simulink model "OldCameraGantryStuff"  (Simulink 7.8)
settings: Solver=FixedStepDiscrete  SolverMode=SingleTasking  StartTime=0.0  StopTime=5.659  FixedStep=0.001  RelTol=1e-3
values from neighbouring files (symbols this model uses):
  T_step = 0.01    [CoefficientsForFilters.mat]    (also in matlab.mat = 0.001)
undefined symbols (not defined in the file or in its folder): DiscIntNeverNeededParam
settings Model: Creator=Marx  LastModifiedBy=root
settings OptimizationCC: OptimizeModelRefInitCode=on  LifeSpan=1
settings HardwareCC: ProdBitPerInt=16  ProdBitPerPointer=16  ProdEndianess=LittleEndian  ProdWordSize=16  ProdHWDeviceType=16-bit Generic
settings RTWCC: SystemTargetFile=dspic.tlc  GenCodeOnly=on  MakeCommand=make_CreateMPLAB  TemplateMakefile=dspic_pic30_gcc.tmf  PostCodeGenCommand=dsPIC_Compile()  Description=Embedded Target for Microchip dsPIC (real-time)  ProcessScript=dspic_make_rtw_hook
settings CodeAppCC: IgnoreCustomStorageClasses=off
settings STFCustomTargetCC: IncludeMdlTerminateFcn=off  GeneratePreprocessorConditionals=Use local settings  CombineOutputUpdateFcns=on  SuppressErrorStatus=on  ERTCustomFileBanners=on  SupportContinuousTime=off  SupportNonInlinedSFcns=off  SystemTargetFile=dspic.tlc
settings ERTTargetCC: MultiwordLength=2048  ParMdlRefBuildCompliant=off  CompOptLevelCompliant=off  ConcurrentExecutionCompliant=off  IncludeMdlTerminateFcn=off  SuppressErrorStatus=on  ERTFirstTimeCompliant=off  ModelStepFunctionPrototypeControlCompliant=off  CPPClassGenCompliant=off  ExtModeMexFile=noextcomm  InlinedParameterPlacement=NonHierarchical  ERTSrcFileBannerTemplate=dsPIC_code_template.cgt  ERTHdrFileBannerTemplate=dsPIC_code_template.cgt  ERTDataSrcFileTemplate=dsPIC_code_template.cgt  ERTDataHdrFileTemplate=dsPIC_code_template.cgt  ERTCustomFileTemplate=dsPIC_main.tlc  ConvertIfToSwitch=off  SuppressUnreachableDefaultCases=off
settings CustomProperty: DataType=string  Value=C:\PROGRA~1\MATLAB\R2011b\bin\win64\gmake

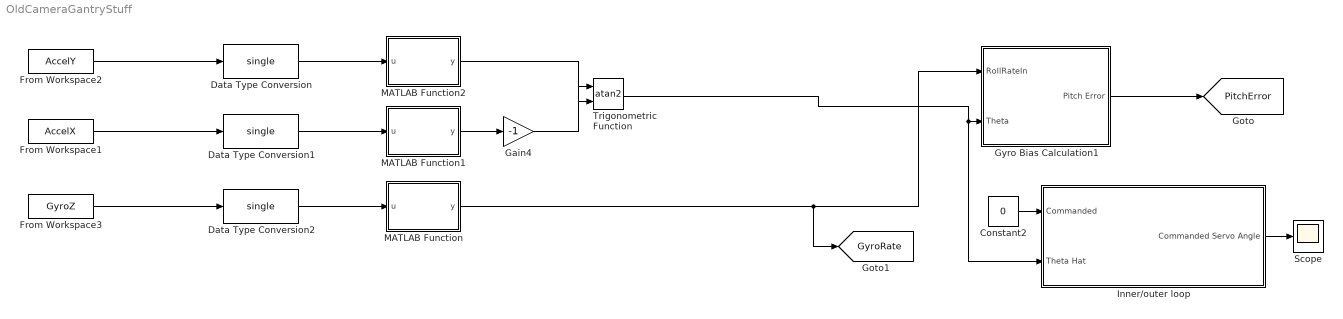
== system OldCameraGantryStuff ==
  Constant2 : Constant  Value=0
  Data Type Conversion : DataTypeConversion  OutMax=4095  OutDataTypeStr=single
  Data Type Conversion1 : DataTypeConversion  OutMax=4095  OutDataTypeStr=single
  Data Type Conversion2 : DataTypeConversion  OutMax=4095  OutDataTypeStr=single  RndMeth=Simplest
  From Workspace1 : FromWorkspace  VariableName=AccelX  SampleTime=.001
  From Workspace2 : FromWorkspace  VariableName=AccelY  SampleTime=.001
  From Workspace3 : FromWorkspace  VariableName=GyroZ  SampleTime=.001
  Gain4 : Gain  Gain=-1
  Gyro Bias Calculation1 : Subsystem
  Inner/outer loop : Subsystem
  MATLAB Function : MATLAB Function  TreatAsAtomicUnit=on
  MATLAB Function1 : MATLAB Function  TreatAsAtomicUnit=on
  MATLAB Function2 : MATLAB Function  TreatAsAtomicUnit=on
  Scope : Scope
  Trigonometric Function : Trigonometry  Operator=atan2
  tag scope: GyroRate=global, PitchError=global
  wires:
  Constant2/1 -> Inner/outer loop/1(Commanded)
  Gyro Bias Calculation1/1(Pitch Error) -> [PitchError]
  Data Type Conversion2/1 -> MATLAB Function/1(u)
  Trigonometric Function/1 -> Gyro Bias Calculation1/2(Theta), Inner/outer loop/2(Theta Hat)
  Gain4/1 -> Trigonometric Function/1
  From Workspace1/1 -> Data Type Conversion1/1
  From Workspace2/1 -> Data Type Conversion/1
  From Workspace3/1 -> Data Type Conversion2/1
  Inner/outer loop/1(Commanded Servo Angle) -> Scope/1
  Data Type Conversion1/1 -> MATLAB Function1/1(u)
  Data Type Conversion/1 -> MATLAB Function2/1(u)
  MATLAB Function/1(y) -> Gyro Bias Calculation1/1(RollRateIn), [GyroRate]
  MATLAB Function1/1(y) -> Gain4/1
  MATLAB Function2/1(y) -> Trigonometric Function/2

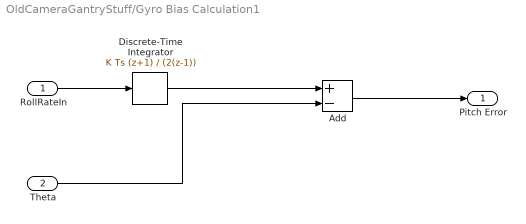
== system OldCameraGantryStuff/Gyro Bias Calculation1 ==
  RollRateIn : Inport
  Theta : Inport  Port=2
  Add : Sum  Inputs=+-
  Discrete-Time Integrator : DiscreteIntegrator  IntegratorMethod=Integration: Trapezoidal  SampleTime=T_step  UpperSaturationLimit=1  LowerSaturationLimit=-1  ICPrevOutput=DiscIntNeverNeededParam  ICPrevScaledInput=DiscIntNeverNeededParam
  Pitch Error : Outport
  wires:
  RollRateIn/1 -> Discrete-Time Integrator/1
  Add/1 -> Pitch Error/1
  Discrete-Time Integrator/1 -> Add/1
  Theta/1 -> Add/2

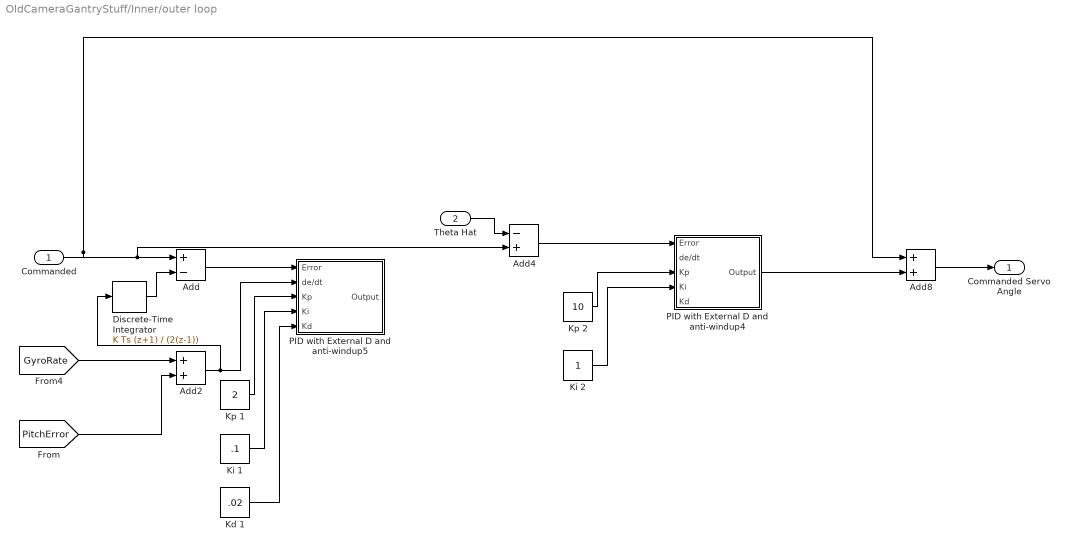
== system OldCameraGantryStuff/Inner/outer loop ==
  Commanded : Inport
  Theta Hat : Inport  Port=2
  Add : Sum  Inputs=+-
  Add2 : Sum
  Add4 : Sum  Inputs=-+
  Add8 : Sum
  Discrete-Time Integrator : DiscreteIntegrator  IntegratorMethod=Integration: Trapezoidal  SampleTime=T_step  ICPrevOutput=DiscIntNeverNeededParam  ICPrevScaledInput=DiscIntNeverNeededParam
  Kd 1 : Constant  Value=.02
  Ki 1 : Constant  Value=.1
  Ki 2 : Constant
  Kp 1 : Constant  Value=2
  Kp 2 : Constant  Value=10
  PID with External D and anti-windup4 : Subsystem
  PID with External D and anti-windup5 : Subsystem
  Commanded Servo Angle : Outport
  wires:
  Add8/1 -> Commanded Servo Angle/1
  Commanded/1 -> Add8/1, Add/1, Add4/2
  Add2/1 -> PID with External D and anti-windup5/2(de/dt), Discrete-Time Integrator/1
  Kp 1/1 -> PID with External D and anti-windup5/3(Kp)
  Ki 1/1 -> PID with External D and anti-windup5/4(Ki)
  Kd 1/1 -> PID with External D and anti-windup5/5(Kd)
  Add4/1 -> PID with External D and anti-windup4/1(Error)
  Kp 2/1 -> PID with External D and anti-windup4/3(Kp)
  Ki 2/1 -> PID with External D and anti-windup4/4(Ki)
  [PitchError] -> Add2/2
  [GyroRate] -> Add2/1
  Theta Hat/1 -> Add4/1
  PID with External D and anti-windup4/1(Output) -> Add8/2
  Add/1 -> PID with External D and anti-windup5/1(Error)
  Discrete-Time Integrator/1 -> Add/2

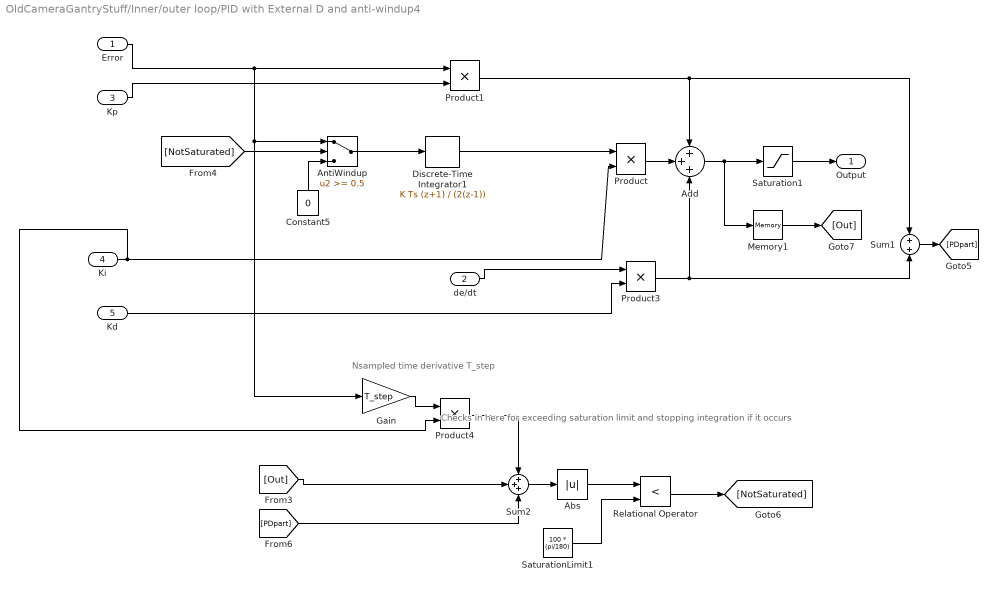
== system OldCameraGantryStuff/Inner/outer loop/PID with External D and anti-windup4 ==
  note: Nsampled time derivative
      | T_step
  note: Checks in here for
      | exceeding saturation
      | limit and stopping
      | integration if it occurs
  Error : Inport
  de/dt : Inport  Port=2
  Kp : Inport  Port=3
  Ki : Inport  Port=4
  Kd : Inport  Port=5
  Abs : Abs
  Add : Sum  Inputs=+++
  AntiWindup : Switch  Threshold=0.5
  Constant5 : Constant  Value=0  OutDataTypeStr=double
  Discrete-Time Integrator1 : DiscreteIntegrator  IntegratorMethod=Integration: Trapezoidal  SampleTime=T_step  ICPrevOutput=DiscIntNeverNeededParam  ICPrevScaledInput=DiscIntNeverNeededParam
  Gain : Gain  Gain=T_step
  Memory1 : Memory  InheritSampleTime=on
  Product{,1,3..4} (4 alike) : Product  RndMeth=Zero
  Relational Operator : RelationalOperator  Operator=<  OutDataTypeStr=boolean
  Saturation1 : Saturate  UpperLimit=100 * (pi/180)  LowerLimit=-100 * (pi/180)
  SaturationLimit1 : Constant  Value=100 * (pi/180)
  Sum1 : Sum  Inputs=+|+
  Sum2 : Sum  Inputs=+++
  Output : Outport
  wires:
  [NotSaturated] -> AntiWindup/2
  Abs/1 -> Relational Operator/1
  SaturationLimit1/1 -> Relational Operator/2
  Saturation1/1 -> Output/1
  Product3/1 -> Add/3, Sum1/2
  de/dt/1 -> Product3/1
  Kd/1 -> Product3/2
  Add/1 -> Memory1/1, Saturation1/1
  Product1/1 -> Sum1/1, Add/1
  Product/1 -> Add/2
  Kp/1 -> Product1/2
  Discrete-Time Integrator1/1 -> Product/1
  Ki/1 -> Product/2, Product4/2
  Error/1 -> Product1/1, AntiWindup/1, Gain/1
  AntiWindup/1 -> Discrete-Time Integrator1/1
  Constant5/1 -> AntiWindup/3
  Sum1/1 -> [PDpart]
  [Out] -> Sum2/2
  Sum2/1 -> Abs/1
  Gain/1 -> Product4/1
  Product4/1 -> Sum2/1
  Memory1/1 -> [Out]
  [PDpart] -> Sum2/3
  Relational Operator/1 -> [NotSaturated]

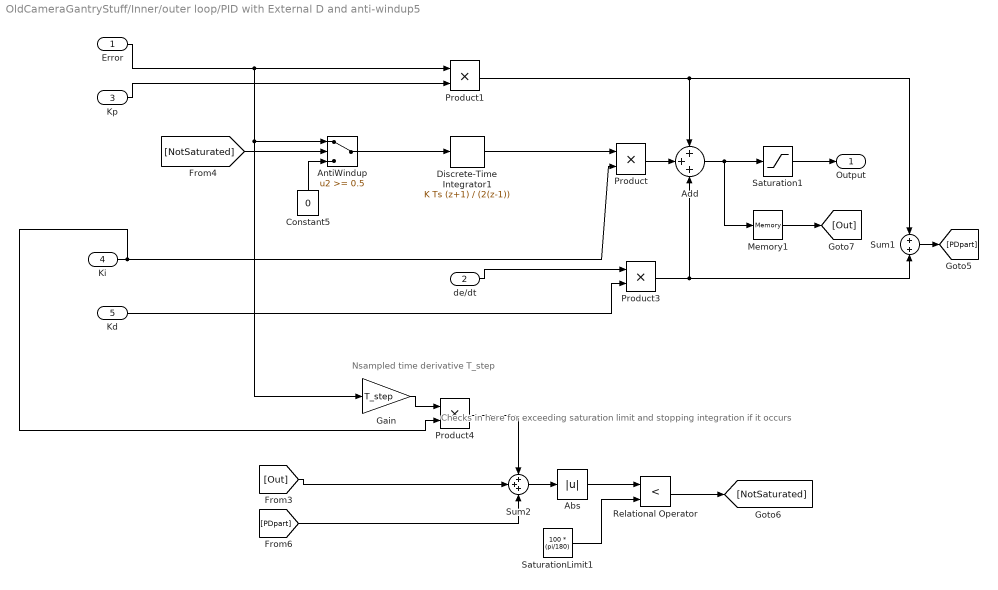
== system OldCameraGantryStuff/Inner/outer loop/PID with External D and anti-windup5 ==
  note: Nsampled time derivative
      | T_step
  note: Checks in here for
      | exceeding saturation
      | limit and stopping
      | integration if it occurs
  Error : Inport
  de/dt : Inport  Port=2
  Kp : Inport  Port=3
  Ki : Inport  Port=4
  Kd : Inport  Port=5
  Abs : Abs
  Add : Sum  Inputs=+++
  AntiWindup : Switch  Threshold=0.5
  Constant5 : Constant  Value=0  OutDataTypeStr=double
  Discrete-Time Integrator1 : DiscreteIntegrator  IntegratorMethod=Integration: Trapezoidal  SampleTime=T_step  ICPrevOutput=DiscIntNeverNeededParam  ICPrevScaledInput=DiscIntNeverNeededParam
  Gain : Gain  Gain=T_step
  Memory1 : Memory  InheritSampleTime=on
  Product{,1,3..4} (4 alike) : Product  RndMeth=Zero
  Relational Operator : RelationalOperator  Operator=<  OutDataTypeStr=boolean
  Saturation1 : Saturate  UpperLimit=100 * (pi/180)  LowerLimit=-100 * (pi/180)
  SaturationLimit1 : Constant  Value=100 * (pi/180)
  Sum1 : Sum  Inputs=+|+
  Sum2 : Sum  Inputs=+++
  Output : Outport
  wires:
  [NotSaturated] -> AntiWindup/2
  Abs/1 -> Relational Operator/1
  SaturationLimit1/1 -> Relational Operator/2
  Saturation1/1 -> Output/1
  Product3/1 -> Add/3, Sum1/2
  de/dt/1 -> Product3/1
  Kd/1 -> Product3/2
  Add/1 -> Memory1/1, Saturation1/1
  Product1/1 -> Sum1/1, Add/1
  Product/1 -> Add/2
  Kp/1 -> Product1/2
  Discrete-Time Integrator1/1 -> Product/1
  Ki/1 -> Product/2, Product4/2
  Error/1 -> Product1/1, AntiWindup/1, Gain/1
  AntiWindup/1 -> Discrete-Time Integrator1/1
  Constant5/1 -> AntiWindup/3
  Sum1/1 -> [PDpart]
  [Out] -> Sum2/2
  Sum2/1 -> Abs/1
  Gain/1 -> Product4/1
  Product4/1 -> Sum2/1
  Memory1/1 -> [Out]
  [PDpart] -> Sum2/3
  Relational Operator/1 -> [NotSaturated]

== matlab function MATLAB Function1 ==
  data: u input double; y output double
function y = fcn(u)
%#codegen

y = u/32.8;

== matlab function MATLAB Function ==
  data: u input double; y output double
function y = fcn(u)
%#codegen

y = ((u/131) * (pi/180));

== matlab function MATLAB Function2 ==
  data: u input double; y output double
function y = fcn(u)
%#codegen

y = u/32.8;
